simulink model "test_model"  (R2020a)
settings: Solver=FixedStepDiscrete  StartTime=0.0  StopTime=38  FixedStep=1e-3  RelTol=1e-3  EnableMultiTasking=on
settings Model: Creator=nori_ohta  LastModifiedBy=103544
settings DataIOCC: SaveFormat=Array  SaveOutput=off  SignalLogging=off  DSMLogging=off  VisualizeSimOutput=off  SaveTime=off  ReturnWorkspaceOutputs=off
settings OptimizationCC: LifeSpan=inf
settings DebuggingCC: SFUnexpectedBacktrackingDiag=warning  SFNoUnconditionalDefaultTransitionDiag=warning  SFExecutionAtInitializationDiag=none  ArithmeticOperatorsInVariantConditions=warning
settings HardwareCC: ProdBitPerPointer=32  ProdBitPerSizeT=32  ProdBitPerPtrDiffT=32  ProdLargestAtomicFloat=None  ProdIntDivRoundTo=Undefined  ProdEndianess=Unspecified  ProdWordSize=32  ProdHWDeviceType=32-bit Generic
settings ModelReferenceCC: PropagateSignalLabelsOutOfModel=off
settings SFSimCC: SimUseLocalCustomCode=off  CustomCodeUndefinedFunction=UseInterfaceOnly
settings RTWCC: RTWUseLocalCustomCode=off
settings CodeAppCC: StateflowObjectComments=on
settings GRTTargetCC: TargetLangStandard=C89/C90 (ANSI)
settings ConfigComp: CovMetricSettings=dw  CovHtmlReporting=on  CovSaveCumulativeToWorkspaceVar=on  CovSaveSingleToWorkspaceVar=on  CovExternalEMLEnable=off

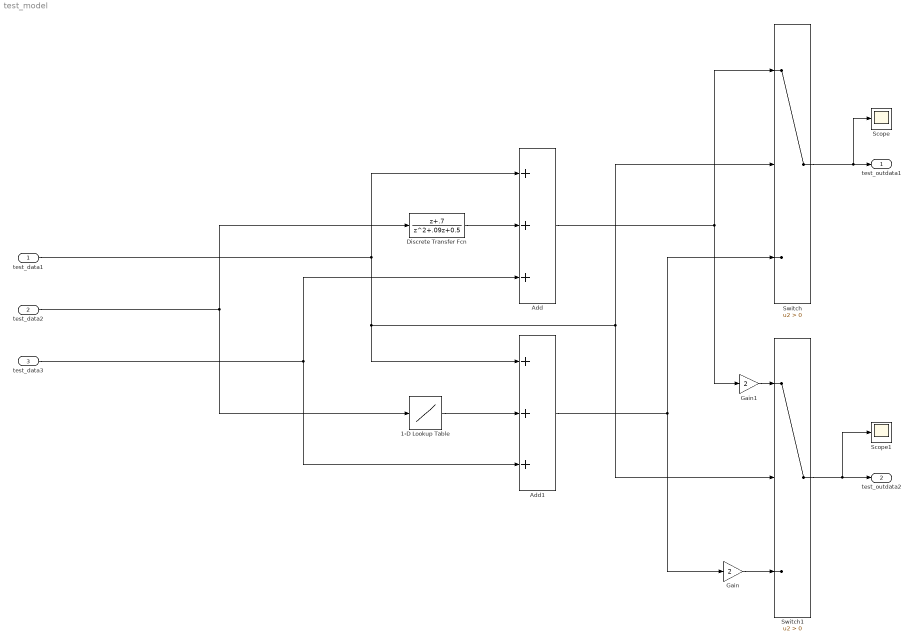
== system test_model ==
  test_data1 : Inport
  test_data2 : Inport  Port=2
  test_data3 : Inport  Port=3
  1-D Lookup Table : Lookup_n-D  NumberOfTableDimensions=1  BreakpointsForDimension1=[-5:5]  Table=tanh([-5:5])  InputSameDT=on
  Add : Sum  Inputs=+++
  Add1 : Sum  Inputs=+++  SampleTime=.01
  Discrete Transfer Fcn : DiscreteTransferFcn  Numerator=[1 .7]  Denominator=[1 .09 0.5]  SampleTime=.01
  Gain : Gain  Gain=2
  Gain1 : Gain  Gain=2
  Scope : Scope
  Scope1 : Scope
  Switch : Switch  Criteria=u2 > Threshold
  Switch1 : Switch  Criteria=u2 > Threshold
  test_outdata1 : Outport
  test_outdata2 : Outport  Port=2
  wires:
  Switch/1 -> Scope/1, test_outdata1/1
  Add/1 -> Switch/1, Gain1/1
  Add1/1 -> Switch/3, Gain/1
  Switch1/1 -> Scope1/1, test_outdata2/1
  Discrete Transfer Fcn/1 -> Add/2
  test_data3/1 -> Add1/3, Add/3
  1-D Lookup Table/1 -> Add1/2
  test_data2/1 -> 1-D Lookup Table/1, Discrete Transfer Fcn/1
  test_data1/1 -> Add/1, Switch/2, Switch1/2, Add1/1
  Gain/1 -> Switch1/3
  Gain1/1 -> Switch1/1
